simulink model "week1_problem7"  (R2020b)
settings: Solver=VariableStepAuto  StartTime=0.0  StopTime=10.0  RelTol=1e-3
libraries: simulink x1
settings Model: Creator=sai  LastModifiedBy=sai

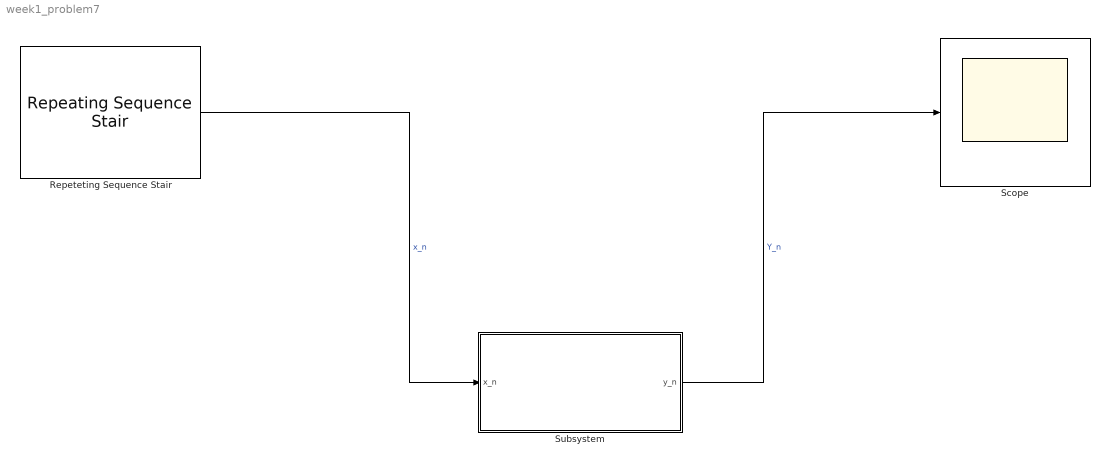
== system week1_problem7 ==
  Repeteting Sequence Stair : simulink/Sources/Repeating Sequence Stair  OutValues=[1 0 1 0 1 0 0 0 1 0 1 1].'  tsamp=-1  OutMin=[]  OutMax=[]  OutDataTypeStr=double  OutputDataTypeScalingMode=double  OutDataType=fixdt(0,8)  ConRadixGroup=Best Precision: Vector-wise  OutScaling=2^-12
  Scope : Scope
  Subsystem : Subsystem
  wires:
  Repeteting Sequence Stair/1 -> Subsystem/1(x_n)  "x_n"
  Subsystem/1(y_n) -> Scope/1  "Y_n"

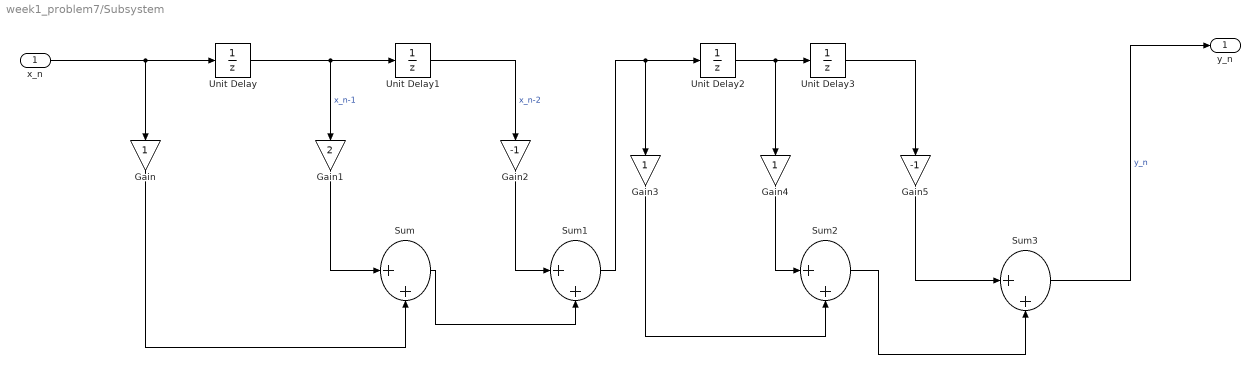
== system week1_problem7/Subsystem ==
  x_n : Inport  OutDataTypeStr=double  PortDimensions=1  SampleTime=[0.20000000000000001,0]
  Gain : Gain
  Gain1 : Gain  Gain=2
  Gain2 : Gain  Gain=-1
  Gain3 : Gain
  Gain4 : Gain
  Gain5 : Gain  Gain=-1
  Sum{,1..3} (4 alike) : Sum  Inputs=|++
  Unit Delay{,1..3} (4 alike) : UnitDelay  SampleTime=-1  HasFrameUpgradeWarning=on
  y_n : Outport  OutDataTypeStr=double  PortDimensions=1  SampleTime=[0.20000000000000001,0]
  wires:
  Unit Delay/1 -> Unit Delay1/1, Gain1/1  "x_n-1"
  Unit Delay1/1 -> Gain2/1  "x_n-2"
  Unit Delay2/1 -> Unit Delay3/1, Gain4/1
  Gain/1 -> Sum/2
  Sum/1 -> Sum1/2
  Gain4/1 -> Sum2/1
  Unit Delay3/1 -> Gain5/1
  Sum1/1 -> Gain3/1, Unit Delay2/1
  Gain3/1 -> Sum2/2
  Gain2/1 -> Sum1/1
  Sum3/1 -> y_n/1  "y_n"
  x_n/1 -> Unit Delay/1, Gain/1
  Sum2/1 -> Sum3/2
  Gain1/1 -> Sum/1
  Gain5/1 -> Sum3/1
